simulink model "MODEL"  (R2019b)
settings: Solver=ode1  StartTime=0.0  StopTime=50  FixedStep=0.001  RelTol=1e-3  EnableMultiTasking=on
PreLoadFcn:
  | run('m-files/add_to_path.m')
InitFcn:
  | create_ephysenet_inifile
undefined symbols (not defined in the file or in its folder): car
libraries: car_library x1
CloseFcn:
  | delete_ephysenet_inifile
settings Model: Creator=ciba  LastModifiedBy=LongLongMagnumDong
settings SolverCC: AutoInsertRateTranBlk=on
settings DataIOCC: LimitDataPoints=on  SaveFormat=Structure  SaveState=on  SignalLogging=off  ReturnWorkspaceOutputs=off
settings OptimizationCC: LifeSpan=inf
settings DebuggingCC: SolverPrmCheckMsg=warning  SFUnexpectedBacktrackingDiag=warning  SFNoUnconditionalDefaultTransitionDiag=warning  SFExecutionAtInitializationDiag=none  ArithmeticOperatorsInVariantConditions=warning
settings HardwareCC: ProdBitPerPointer=32  ProdBitPerSizeT=32  ProdBitPerPtrDiffT=32  ProdLargestAtomicFloat=None  ProdIntDivRoundTo=Undefined  ProdEndianess=Unspecified  ProdWordSize=32  ProdHWDeviceType=32-bit Generic
settings ModelReferenceCC: PropagateSignalLabelsOutOfModel=off
settings SFSimCC: SimUseLocalCustomCode=off  CustomCodeUndefinedFunction=UseInterfaceOnly
settings RTWCC: RTWUseLocalCustomCode=off
settings CodeAppCC: StateflowObjectComments=on
settings GRTTargetCC: TargetLangStandard=C89/C90 (ANSI)  GeneratePreprocessorConditionals=Disable all
settings ConfigComp: CovMetricSettings=dw  CovHtmlReporting=on  CovSaveCumulativeToWorkspaceVar=on  CovSaveSingleToWorkspaceVar=on  CovExternalEMLEnable=off

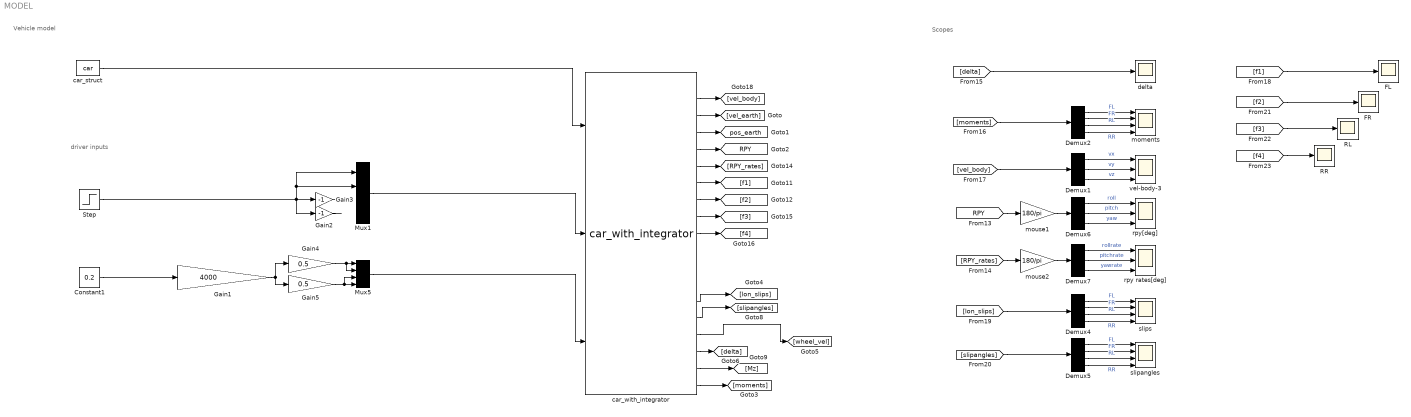
== system MODEL ==
  note: driver inputs
  note: Scopes
  note: Vehicle model
  Constant1 : Constant  Value=0.2
  Demux1 : Demux  Outputs=3
  Demux2 : Demux
  Demux4 : Demux
  Demux5 : Demux
  Demux6 : Demux  Outputs=3
  Demux7 : Demux  Outputs=3
  FL : Scope
  FR : Scope
  Gain1 : Gain  Gain=4000
  Gain2 : Gain  Gain=-1
  Gain3 : Gain  Gain=-1
  Gain4 : Gain  Gain=0.5
  Gain5 : Gain  Gain=0.5
  Mux1 : Mux
  Mux5 : Mux
  RL : Scope
  RR : Scope
  Step : Step  Time=10  After=deg2rad(15)  SampleTime=0
  car_struct : Constant  Value=car  OutDataTypeStr=Bus: car_bus
  car_with_integrator : car_library/car_with_integrator  SystemSampleTime=-1  Latency=0  AutoFrameSizeCalculation=off
      link override Constant2: Value=[1;1;1;1]
  delta : Scope
  moments : Scope  NumInputPorts=4
  mouse1 : Gain  Gain=180/pi
  mouse2 : Gain  Gain=180/pi
  rpy rates[deg] : Scope  NumInputPorts=3
  "rpy[deg] " : Scope  NumInputPorts=3
  slipangles : Scope  NumInputPorts=4
  slips : Scope  NumInputPorts=4
  "vel-body-3 " : Scope  NumInputPorts=3
  tag scope: RPY=global, pos_earth=global
  wires:
  car_with_integrator/3 -> [vel_earth]
  car_with_integrator/4 -> [pos_earth]
  car_with_integrator/16 -> [wheel_vel]
  car_with_integrator/15 -> [slipangles]
  car_with_integrator/5 -> [RPY]
  car_with_integrator/19 -> [moments]
  car_with_integrator/17 -> [delta]
  [RPY] -> mouse1/1
  [delta] -> delta/1
  car_with_integrator/6 -> [RPY_rates]
  [moments] -> Demux2/1
  Demux2/1 -> moments/1  "FL"
  Demux2/2 -> moments/2  "FR"
  Demux2/3 -> moments/3  "RL"
  Demux2/4 -> moments/4  "RR"
  Demux4/1 -> slips/1  "FL"
  Demux4/2 -> slips/2  "FR"
  Demux4/3 -> slips/3  "RL"
  Demux4/4 -> slips/4  "RR"
  [lon_slips] -> Demux4/1
  Demux5/1 -> slipangles/1  "FL"
  Demux5/2 -> slipangles/2  "FR"
  Demux5/3 -> slipangles/3  "RL"
  Demux5/4 -> slipangles/4  "RR"
  [slipangles] -> Demux5/1
  car_with_integrator/14 -> [lon_slips]
  car_with_integrator/18 -> [Mz]
  car_with_integrator/7 -> [f1]
  car_with_integrator/8 -> [f2]
  car_with_integrator/9 -> [f3]
  car_with_integrator/10 -> [f4]
  Step/1 -> Mux1/2, Mux1/1, Gain2/1, Gain3/1
  Mux5/1 -> car_with_integrator/3
  Gain1/1 -> Gain4/1, Gain5/1
  Gain5/1 -> Mux5/4, Mux5/3
  Gain4/1 -> Mux5/2, Mux5/1
  car_struct/1 -> car_with_integrator/1
  Gain2/1 -> ?
  Gain3/1 -> ?
  car_with_integrator/2 -> [vel_body]
  [vel_body] -> Demux1/1
  Demux1/2 -> "vel-body-3 "/2  "vy"
  Demux1/1 -> "vel-body-3 "/1  "vx"
  Demux1/3 -> "vel-body-3 "/3  "vz"
  Constant1/1 -> Gain1/1
  Mux1/1 -> car_with_integrator/2
  mouse1/1 -> Demux6/1
  Demux6/1 -> "rpy[deg] "/1  "roll"
  Demux6/2 -> "rpy[deg] "/2  "pitch"
  Demux6/3 -> "rpy[deg] "/3  "yaw"
  Demux7/3 -> rpy rates[deg]/3  "yawrate"
  Demux7/2 -> rpy rates[deg]/2  "pitchrate"
  [RPY_rates] -> mouse2/1
  mouse2/1 -> Demux7/1
  Demux7/1 -> rpy rates[deg]/1  "rollrate"
  [f1] -> FL/1
  [f2] -> FR/1
  [f3] -> RL/1
  [f4] -> RR/1
